simulink model "Autotrans_shift"  (R2024b)
settings: Solver=VariableStepAuto  StartTime=0.0  StopTime=35.0  FixedStep=0.001  RelTol=0.001
model workspace (MATLAB code in the model file):
  | load sldemo_autotrans_data; %load initial conditions and other necessary data
undefined symbols (not defined in the file or in its folder): converter_data, downtab, emap, Hecate_brake1, Hecate_brake2, Hecate_throttle1, Hecate_throttle2, Hecate_trans, Iei, uptab, vehicledata
(part 2 of 2)

== stateflow chart Autotrans_shift/RequirementsTable2 ==
  (default) -> (junction 1073745136)
  (junction 1073745136) -> (junction 1073745137) : {
      | % SF_REQ_REV_07
      | }
  (junction 1073745137) -> (junction 1073745139) : {
      | % ExcEvals:
      | % PriEvals:
      | }
  (junction 1073745139) -> (junction 1073745141) : {
      | % HEADER_ASSIGNMENTS
      |
      | }
  (junction 1073745141) -> (junction 1073745143) : {
      | % START_A_4
      | }
  (junction 1073745143) -> (junction 1073745145) : {
      | }
  (junction 1073745145) -> (junction 1073745147)
  (junction 1073745147) -> (junction 1073745149) : {
      | }
  (junction 1073745149) -> (junction 1073745151) : {
      | % END_A_4
      | }
  (junction 1073745151) -> (junction 1073745153) : {
      | % START_R_7
      | }
  (junction 1073745153) -> (junction 1073745155) : {
      | }
  (junction 1073745155) -> (junction 1073745157)
  (junction 1073745157) -> (junction 1073745159) [order 1] : [(((t) >= (0) && (t) <= (20)))]
  (junction 1073745157) -> (junction 1073745165) [order 2]
  (junction 1073745159) -> (junction 1073745161) : {
      | reqtable_postcondition(((speed2)/115 < 1), 'R:1');
      |
      |
      |
      |
      | }
  (junction 1073745161) -> (junction 1073745163) : {
      | }
  (junction 1073745163) -> (junction 1073745165)
  (junction 1073745165) -> (junction 1073745167)
  (junction 1073745167) -> (junction 1073745169) : {
      | % END_R_7
      | }
  (junction 1073745169) -> (junction 1073745171) : {
      | % START_R_19
      | }
  (junction 1073745171) -> (junction 1073745173) : {
      | }
  (junction 1073745173) -> (junction 1073745175)
  (junction 1073745175) -> (junction 1073745177) [order 1] : [(((t) >= (0) && (t) <= (10)))]
  (junction 1073745175) -> (junction 1073745183) [order 2]
  (junction 1073745177) -> (junction 1073745179) : {
      | reqtable_postcondition(((RPM2)/4800 < 1), 'R:2');
      |
      |
      |
      |
      | }
  (junction 1073745179) -> (junction 1073745181) : {
      | }
  (junction 1073745181) -> (junction 1073745183)
  (junction 1073745183) -> (junction 1073745185)
  (junction 1073745185) -> (junction 1073745187) : {
      | % END_R_19
      | }
  (junction 1073745187) -> (junction 1073745189) : {
      | % START_R_34
      | }
  (junction 1073745189) -> (junction 1073745191) : {
      | }
  (junction 1073745191) -> (junction 1073745193)
  (junction 1073745193) -> (junction 1073745195) [order 1] : [((t)== 0)]
  (junction 1073745193) -> (junction 1073745201) [order 2]
  (junction 1073745195) -> (junction 1073745197) : {
      | flaga_out = true;
      | flagb_out = true;
      | flagc_out = true;
      |
      | }
  (junction 1073745197) -> (junction 1073745199) : {
      | }
  (junction 1073745199) -> (junction 1073745201)
  (junction 1073745201) -> (junction 1073745203)
  (junction 1073745203) -> (junction 1073745205) : {
      | % END_R_34
      | }
  (junction 1073745205) -> (junction 1073745207) : {
      | % START_R_22
      | }
  (junction 1073745207) -> (junction 1073745209) : {
      | }
  (junction 1073745209) -> (junction 1073745211)
  (junction 1073745211) -> (junction 1073745213) [order 1] : [(((t) <= (4))) && (speed1 >= 35)]
  (junction 1073745211) -> (junction 1073745219) [order 2]
  (junction 1073745213) -> (junction 1073745215) : {
      | flaga_out = false
      |
      |
      |
      | }
  (junction 1073745215) -> (junction 1073745217) : {
      | }
  (junction 1073745217) -> (junction 1073745219)
  (junction 1073745219) -> (junction 1073745221)
  (junction 1073745221) -> (junction 1073745223) : {
      | % END_R_22
      | }
  (junction 1073745223) -> (junction 1073745225) : {
      | % START_R_67
      | }
  (junction 1073745225) -> (junction 1073745227) : {
      | }
  (junction 1073745227) -> (junction 1073745229)
  (junction 1073745229) -> (junction 1073745231) [order 1] : [((t)> 4 || ((t)> 0 && speed1 < 35))]
  (junction 1073745229) -> (junction 1073745237) [order 2]
  (junction 1073745231) -> (junction 1073745233) : {
      | flaga_out = prev(flaga_out);
      |
      |
      |
      | }
  (junction 1073745233) -> (junction 1073745235) : {
      | }
  (junction 1073745235) -> (junction 1073745237)
  (junction 1073745237) -> (junction 1073745239)
  (junction 1073745239) -> (junction 1073745241) : {
      | % END_R_67
      | }
  (junction 1073745241) -> (junction 1073745243) : {
      | % START_R_52
      | }
  (junction 1073745243) -> (junction 1073745245) : {
      | }
  (junction 1073745245) -> (junction 1073745247)
  (junction 1073745247) -> (junction 1073745249) [order 1] : [duration((((t) <= (30))) && (RPM1 < 3000)) >= 30]
  (junction 1073745247) -> (junction 1073745255) [order 2]
  (junction 1073745249) -> (junction 1073745251) : {
      | reqtable_postcondition((((flaga_in) == (true))), 'R:6');
      |
      |
      |
      |
      | }
  (junction 1073745251) -> (junction 1073745253) : {
      | }
  (junction 1073745253) -> (junction 1073745255)
  (junction 1073745255) -> (junction 1073745257)
  (junction 1073745257) -> (junction 1073745259) : {
      | % END_R_52
      | }
  (junction 1073745259) -> (junction 1073745261) : {
      | % START_R_16
      | }
  (junction 1073745261) -> (junction 1073745263) : {
      | }
  (junction 1073745263) -> (junction 1073745265)
  (junction 1073745265) -> (junction 1073745267) [order 1] : [(((t) <= (8))) && (speed1 >= 52)]
  (junction 1073745265) -> (junction 1073745273) [order 2]
  (junction 1073745267) -> (junction 1073745269) : {
      |
      | flagb_out = false;
      |
      |
      | }
  (junction 1073745269) -> (junction 1073745271) : {
      | }
  (junction 1073745271) -> (junction 1073745273)
  (junction 1073745273) -> (junction 1073745275)
  (junction 1073745275) -> (junction 1073745277) : {
      | % END_R_16
      | }
  (junction 1073745277) -> (junction 1073745279) : {
      | % START_R_70
      | }
  (junction 1073745279) -> (junction 1073745281) : {
      | }
  (junction 1073745281) -> (junction 1073745283)
  (junction 1073745283) -> (junction 1073745285) [order 1] : [((t)> 8 || ((t)> 0 && speed1 < 52))]
  (junction 1073745283) -> (junction 1073745291) [order 2]
  (junction 1073745285) -> (junction 1073745287) : {
      |
      | flagb_out = prev(flagb_out);
      |
      |
      | }
  (junction 1073745287) -> (junction 1073745289) : {
      | }
  (junction 1073745289) -> (junction 1073745291)
  (junction 1073745291) -> (junction 1073745293)
  (junction 1073745293) -> (junction 1073745295) : {
      | % END_R_70
      | }
  (junction 1073745295) -> (junction 1073745297) : {
      | % START_R_55
      | }
  (junction 1073745297) -> (junction 1073745299) : {
      | }
  (junction 1073745299) -> (junction 1073745301)
  (junction 1073745301) -> (junction 1073745303) [order 1] : [duration((((t) <= (30))) && (RPM1 < 2900)) >= 30]
  (junction 1073745301) -> (junction 1073745309) [order 2]
  (junction 1073745303) -> (junction 1073745305) : {
      | reqtable_postcondition((((flagb_in) == (true))), 'R:9');
      |
      |
      |
      |
      | }
  (junction 1073745305) -> (junction 1073745307) : {
      | }
  (junction 1073745307) -> (junction 1073745309)
  (junction 1073745309) -> (junction 1073745311)
  (junction 1073745311) -> (junction 1073745313) : {
      | % END_R_55
      | }
  (junction 1073745313) -> (junction 1073745315) : {
      | % START_R_28
      | }
  (junction 1073745315) -> (junction 1073745317) : {
      | }
  (junction 1073745317) -> (junction 1073745319)
  (junction 1073745319) -> (junction 1073745321) [order 1] : [(((t) <= (20))) && (speed1 >= 65)]
  (junction 1073745319) -> (junction 1073745327) [order 2]
  (junction 1073745321) -> (junction 1073745323) : {
      |
      |
      | flagc_out = false;
      |
      | }
  (junction 1073745323) -> (junction 1073745325) : {
      | }
  (junction 1073745325) -> (junction 1073745327)
  (junction 1073745327) -> (junction 1073745329)
  (junction 1073745329) -> (junction 1073745331) : {
      | % END_R_28
      | }
  (junction 1073745331) -> (junction 1073745333) : {
      | % START_R_73
      | }
  (junction 1073745333) -> (junction 1073745335) : {
      | }
  (junction 1073745335) -> (junction 1073745337)
  (junction 1073745337) -> (junction 1073745339) [order 1] : [((t)> 20 || ((t)> 0 && speed1 < 65))]
  (junction 1073745337) -> (junction 1073745345) [order 2]
  (junction 1073745339) -> (junction 1073745341) : {
      |
      |
      | flagc_out = prev(flagc_out);
      |
      | }
  (junction 1073745341) -> (junction 1073745343) : {
      | }
  (junction 1073745343) -> (junction 1073745345)
  (junction 1073745345) -> (junction 1073745347)
  (junction 1073745347) -> (junction 1073745349) : {
      | % END_R_73
      | }
  (junction 1073745349) -> (junction 1073745351) : {
      | % START_R_58
      | }
  (junction 1073745351) -> (junction 1073745353) : {
      | }
  (junction 1073745353) -> (junction 1073745355)
  (junction 1073745355) -> (junction 1073745357) [order 1] : [duration((((t) <= (30))) && (RPM1 < 3000)) >= 30]
  (junction 1073745355) -> (junction 1073745363) [order 2]
  (junction 1073745357) -> (junction 1073745359) : {
      | reqtable_postcondition((((flagc_in) == (true))), 'R:12');
      |
      |
      |
      |
      | }
  (junction 1073745359) -> (junction 1073745361) : {
      | }
  (junction 1073745361) -> (junction 1073745363)
  (junction 1073745363) -> (junction 1073745365)
  (junction 1073745365) -> (junction 1073745367) : {
      | % END_R_58
      | }
  (junction 1073745367) -> (junction 1073745369) : {
      | % START_R_61
      | }
  (junction 1073745369) -> (junction 1073745371) : {
      | }
  (junction 1073745371) -> (junction 1073745373)
  (junction 1073745373) -> (junction 1073745375) [order 1] : [(((t) >= (0) && (t) <= (50)))]
  (junction 1073745373) -> (junction 1073745381) [order 2]
  (junction 1073745375) -> (junction 1073745377) : {
      | reqtable_postcondition((((speed2) >= (0))) && (((RPM2) >= (0))) && ((flaga_in)== true ||(flaga_in)== false) && ((flagb_in)== true ||(flagb_in)== false) && ((flagc_in)== true ||(flagc_in)== false), 'R:13');
      |
      |
      |
      |
      | }
  (junction 1073745377) -> (junction 1073745379) : {
      | }
  (junction 1073745379) -> (junction 1073745381)
  (junction 1073745381) -> (junction 1073745383)
  (junction 1073745383) -> (junction 1073745385) : {
      | % END_R_61
      | }
  data: RPM1 input; RPM2 input; speed1 input; speed2 input; flaga_out output boolean =true; flagc_out output boolean =true; flagb_out output boolean =true; flaga_in input boolean; flagc_in input boolean; flagb_in input boolean

== stateflow chart Autotrans_shift/RequirementsTable3 ==
  (default) -> (junction 1073745136)
  (junction 1073745136) -> (junction 1073745137) : {
      | % SF_REQ_REV_07
      | }
  (junction 1073745137) -> (junction 1073745139) : {
      | % ExcEvals:
      | % PriEvals:
      | }
  (junction 1073745139) -> (junction 1073745141) : {
      | % HEADER_ASSIGNMENTS
      |
      | }
  (junction 1073745141) -> (junction 1073745143) : {
      | % START_A_4
      | }
  (junction 1073745143) -> (junction 1073745145) : {
      | }
  (junction 1073745145) -> (junction 1073745147)
  (junction 1073745147) -> (junction 1073745149) : {
      | }
  (junction 1073745149) -> (junction 1073745151) : {
      | % END_A_4
      | }
  (junction 1073745151) -> (junction 1073745153) : {
      | % START_R_7
      | }
  (junction 1073745153) -> (junction 1073745155) : {
      | }
  (junction 1073745155) -> (junction 1073745157)
  (junction 1073745157) -> (junction 1073745159) [order 1] : [(((t) >= (0) && (t) <= (25)))]
  (junction 1073745157) -> (junction 1073745165) [order 2]
  (junction 1073745159) -> (junction 1073745161) : {
      | reqtable_postcondition(((speed2)/125 < 1), 'R:1');
      |
      |
      |
      |
      | }
  (junction 1073745161) -> (junction 1073745163) : {
      | }
  (junction 1073745163) -> (junction 1073745165)
  (junction 1073745165) -> (junction 1073745167)
  (junction 1073745167) -> (junction 1073745169) : {
      | % END_R_7
      | }
  (junction 1073745169) -> (junction 1073745171) : {
      | % START_R_19
      | }
  (junction 1073745171) -> (junction 1073745173) : {
      | }
  (junction 1073745173) -> (junction 1073745175)
  (junction 1073745175) -> (junction 1073745177) [order 1] : [(((t) >= (0) && (t) <= (10)))]
  (junction 1073745175) -> (junction 1073745183) [order 2]
  (junction 1073745177) -> (junction 1073745179) : {
      | reqtable_postcondition(((RPM2)/4800 < 1), 'R:2');
      |
      |
      |
      |
      | }
  (junction 1073745179) -> (junction 1073745181) : {
      | }
  (junction 1073745181) -> (junction 1073745183)
  (junction 1073745183) -> (junction 1073745185)
  (junction 1073745185) -> (junction 1073745187) : {
      | % END_R_19
      | }
  (junction 1073745187) -> (junction 1073745189) : {
      | % START_R_34
      | }
  (junction 1073745189) -> (junction 1073745191) : {
      | }
  (junction 1073745191) -> (junction 1073745193)
  (junction 1073745193) -> (junction 1073745195) [order 1] : [((t)== 0)]
  (junction 1073745193) -> (junction 1073745201) [order 2]
  (junction 1073745195) -> (junction 1073745197) : {
      | flaga_out = true;
      | flagb_out = true;
      | flagc_out = true;
      |
      | }
  (junction 1073745197) -> (junction 1073745199) : {
      | }
  (junction 1073745199) -> (junction 1073745201)
  (junction 1073745201) -> (junction 1073745203)
  (junction 1073745203) -> (junction 1073745205) : {
      | % END_R_34
      | }
  (junction 1073745205) -> (junction 1073745207) : {
      | % START_R_22
      | }
  (junction 1073745207) -> (junction 1073745209) : {
      | }
  (junction 1073745209) -> (junction 1073745211)
  (junction 1073745211) -> (junction 1073745213) [order 1] : [(((t) <= (4))) && (speed1 >= 35)]
  (junction 1073745211) -> (junction 1073745219) [order 2]
  (junction 1073745213) -> (junction 1073745215) : {
      | flaga_out = false
      |
      |
      |
      | }
  (junction 1073745215) -> (junction 1073745217) : {
      | }
  (junction 1073745217) -> (junction 1073745219)
  (junction 1073745219) -> (junction 1073745221)
  (junction 1073745221) -> (junction 1073745223) : {
      | % END_R_22
      | }
  (junction 1073745223) -> (junction 1073745225) : {
      | % START_R_67
      | }
  (junction 1073745225) -> (junction 1073745227) : {
      | }
  (junction 1073745227) -> (junction 1073745229)
  (junction 1073745229) -> (junction 1073745231) [order 1] : [((t)> 4 || ((t)> 0 && speed1 < 35))]
  (junction 1073745229) -> (junction 1073745237) [order 2]
  (junction 1073745231) -> (junction 1073745233) : {
      | flaga_out = prev(flaga_out);
      |
      |
      |
      | }
  (junction 1073745233) -> (junction 1073745235) : {
      | }
  (junction 1073745235) -> (junction 1073745237)
  (junction 1073745237) -> (junction 1073745239)
  (junction 1073745239) -> (junction 1073745241) : {
      | % END_R_67
      | }
  (junction 1073745241) -> (junction 1073745243) : {
      | % START_R_52
      | }
  (junction 1073745243) -> (junction 1073745245) : {
      | }
  (junction 1073745245) -> (junction 1073745247)
  (junction 1073745247) -> (junction 1073745249) [order 1] : [duration((((t) <= (30))) && (RPM1 < 3000)) >= 30]
  (junction 1073745247) -> (junction 1073745255) [order 2]
  (junction 1073745249) -> (junction 1073745251) : {
      | reqtable_postcondition((((flaga_in) == (true))), 'R:6');
      |
      |
      |
      |
      | }
  (junction 1073745251) -> (junction 1073745253) : {
      | }
  (junction 1073745253) -> (junction 1073745255)
  (junction 1073745255) -> (junction 1073745257)
  (junction 1073745257) -> (junction 1073745259) : {
      | % END_R_52
      | }
  (junction 1073745259) -> (junction 1073745261) : {
      | % START_R_16
      | }
  (junction 1073745261) -> (junction 1073745263) : {
      | }
  (junction 1073745263) -> (junction 1073745265)
  (junction 1073745265) -> (junction 1073745267) [order 1] : [(((t) <= (8))) && (speed1 >= 50)]
  (junction 1073745265) -> (junction 1073745273) [order 2]
  (junction 1073745267) -> (junction 1073745269) : {
      |
      | flagb_out = false;
      |
      |
      | }
  (junction 1073745269) -> (junction 1073745271) : {
      | }
  (junction 1073745271) -> (junction 1073745273)
  (junction 1073745273) -> (junction 1073745275)
  (junction 1073745275) -> (junction 1073745277) : {
      | % END_R_16
      | }
  (junction 1073745277) -> (junction 1073745279) : {
      | % START_R_70
      | }
  (junction 1073745279) -> (junction 1073745281) : {
      | }
  (junction 1073745281) -> (junction 1073745283)
  (junction 1073745283) -> (junction 1073745285) [order 1] : [((t)> 8 || ((t)> 0 && speed1 < 50))]
  (junction 1073745283) -> (junction 1073745291) [order 2]
  (junction 1073745285) -> (junction 1073745287) : {
      |
      | flagb_out = prev(flagb_out);
      |
      |
      | }
  (junction 1073745287) -> (junction 1073745289) : {
      | }
  (junction 1073745289) -> (junction 1073745291)
  (junction 1073745291) -> (junction 1073745293)
  (junction 1073745293) -> (junction 1073745295) : {
      | % END_R_70
      | }
  (junction 1073745295) -> (junction 1073745297) : {
      | % START_R_55
      | }
  (junction 1073745297) -> (junction 1073745299) : {
      | }
  (junction 1073745299) -> (junction 1073745301)
  (junction 1073745301) -> (junction 1073745303) [order 1] : [duration((((t) <= (30))) && (RPM1 < 3000)) >= 30]
  (junction 1073745301) -> (junction 1073745309) [order 2]
  (junction 1073745303) -> (junction 1073745305) : {
      | reqtable_postcondition((((flagb_in) == (true))), 'R:9');
      |
      |
      |
      |
      | }
  (junction 1073745305) -> (junction 1073745307) : {
      | }
  (junction 1073745307) -> (junction 1073745309)
  (junction 1073745309) -> (junction 1073745311)
  (junction 1073745311) -> (junction 1073745313) : {
      | % END_R_55
      | }
  (junction 1073745313) -> (junction 1073745315) : {
      | % START_R_28
      | }
  (junction 1073745315) -> (junction 1073745317) : {
      | }
  (junction 1073745317) -> (junction 1073745319)
  (junction 1073745319) -> (junction 1073745321) [order 1] : [(((t) <= (20))) && (speed1 >= 67)]
  (junction 1073745319) -> (junction 1073745327) [order 2]
  (junction 1073745321) -> (junction 1073745323) : {
      |
      |
      | flagc_out = false;
      |
      | }
  (junction 1073745323) -> (junction 1073745325) : {
      | }
  (junction 1073745325) -> (junction 1073745327)
  (junction 1073745327) -> (junction 1073745329)
  (junction 1073745329) -> (junction 1073745331) : {
      | % END_R_28
      | }
  (junction 1073745331) -> (junction 1073745333) : {
      | % START_R_73
      | }
  (junction 1073745333) -> (junction 1073745335) : {
      | }
  (junction 1073745335) -> (junction 1073745337)
  (junction 1073745337) -> (junction 1073745339) [order 1] : [((t)> 20 || ((t)> 0 && speed1 < 67))]
  (junction 1073745337) -> (junction 1073745345) [order 2]
  (junction 1073745339) -> (junction 1073745341) : {
      |
      |
      | flagc_out = prev(flagc_out);
      |
      | }
  (junction 1073745341) -> (junction 1073745343) : {
      | }
  (junction 1073745343) -> (junction 1073745345)
  (junction 1073745345) -> (junction 1073745347)
  (junction 1073745347) -> (junction 1073745349) : {
      | % END_R_73
      | }
  (junction 1073745349) -> (junction 1073745351) : {
      | % START_R_58
      | }
  (junction 1073745351) -> (junction 1073745353) : {
      | }
  (junction 1073745353) -> (junction 1073745355)
  (junction 1073745355) -> (junction 1073745357) [order 1] : [duration((((t) <= (30))) && (RPM1 < 2900)) >= 30]
  (junction 1073745355) -> (junction 1073745363) [order 2]
  (junction 1073745357) -> (junction 1073745359) : {
      | reqtable_postcondition((((flagc_in) == (true))), 'R:12');
      |
      |
      |
      |
      | }
  (junction 1073745359) -> (junction 1073745361) : {
      | }
  (junction 1073745361) -> (junction 1073745363)
  (junction 1073745363) -> (junction 1073745365)
  (junction 1073745365) -> (junction 1073745367) : {
      | % END_R_58
      | }
  (junction 1073745367) -> (junction 1073745369) : {
      | % START_R_61
      | }
  (junction 1073745369) -> (junction 1073745371) : {
      | }
  (junction 1073745371) -> (junction 1073745373)
  (junction 1073745373) -> (junction 1073745375) [order 1] : [(((t) >= (0) && (t) <= (50)))]
  (junction 1073745373) -> (junction 1073745381) [order 2]
  (junction 1073745375) -> (junction 1073745377) : {
      | reqtable_postcondition((((speed2) >= (0))) && (((RPM2) >= (0))) && ((flaga_in)== true ||(flaga_in)== false) && ((flagb_in)== true ||(flagb_in)== false) && ((flagc_in)== true ||(flagc_in)== false), 'R:13');
      |
      |
      |
      |
      | }
  (junction 1073745377) -> (junction 1073745379) : {
      | }
  (junction 1073745379) -> (junction 1073745381)
  (junction 1073745381) -> (junction 1073745383)
  (junction 1073745383) -> (junction 1073745385) : {
      | % END_R_61
      | }
  data: RPM1 input; RPM2 input; speed1 input; speed2 input; flaga_out output boolean =true; flagc_out output boolean =true; flagb_out output boolean =true; flaga_in input boolean; flagc_in input boolean; flagb_in input boolean

== stateflow chart Autotrans_shift/RequirementsTable4 ==
  (default) -> (junction 1073745136)
  (junction 1073745136) -> (junction 1073745137) : {
      | % SF_REQ_REV_07
      | }
  (junction 1073745137) -> (junction 1073745139) : {
      | % ExcEvals:
      | % PriEvals:
      | }
  (junction 1073745139) -> (junction 1073745141) : {
      | % HEADER_ASSIGNMENTS
      |
      | }
  (junction 1073745141) -> (junction 1073745143) : {
      | % START_A_4
      | }
  (junction 1073745143) -> (junction 1073745145) : {
      | }
  (junction 1073745145) -> (junction 1073745147)
  (junction 1073745147) -> (junction 1073745149) : {
      | }
  (junction 1073745149) -> (junction 1073745151) : {
      | % END_A_4
      | }
  (junction 1073745151) -> (junction 1073745153) : {
      | % START_R_7
      | }
  (junction 1073745153) -> (junction 1073745155) : {
      | }
  (junction 1073745155) -> (junction 1073745157)
  (junction 1073745157) -> (junction 1073745159) [order 1] : [(((t) >= (0) && (t) <= (25)))]
  (junction 1073745157) -> (junction 1073745165) [order 2]
  (junction 1073745159) -> (junction 1073745161) : {
      | reqtable_postcondition(((speed2)/125 < 1), 'R:1');
      |
      |
      |
      |
      | }
  (junction 1073745161) -> (junction 1073745163) : {
      | }
  (junction 1073745163) -> (junction 1073745165)
  (junction 1073745165) -> (junction 1073745167)
  (junction 1073745167) -> (junction 1073745169) : {
      | % END_R_7
      | }
  (junction 1073745169) -> (junction 1073745171) : {
      | % START_R_19
      | }
  (junction 1073745171) -> (junction 1073745173) : {
      | }
  (junction 1073745173) -> (junction 1073745175)
  (junction 1073745175) -> (junction 1073745177) [order 1] : [(((t) >= (0) && (t) <= (8)))]
  (junction 1073745175) -> (junction 1073745183) [order 2]
  (junction 1073745177) -> (junction 1073745179) : {
      | reqtable_postcondition(((RPM2)/4750 < 1), 'R:2');
      |
      |
      |
      |
      | }
  (junction 1073745179) -> (junction 1073745181) : {
      | }
  (junction 1073745181) -> (junction 1073745183)
  (junction 1073745183) -> (junction 1073745185)
  (junction 1073745185) -> (junction 1073745187) : {
      | % END_R_19
      | }
  (junction 1073745187) -> (junction 1073745189) : {
      | % START_R_34
      | }
  (junction 1073745189) -> (junction 1073745191) : {
      | }
  (junction 1073745191) -> (junction 1073745193)
  (junction 1073745193) -> (junction 1073745195) [order 1] : [((t)== 0)]
  (junction 1073745193) -> (junction 1073745201) [order 2]
  (junction 1073745195) -> (junction 1073745197) : {
      | flaga_out = true;
      | flagb_out = true;
      | flagc_out = true;
      |
      | }
  (junction 1073745197) -> (junction 1073745199) : {
      | }
  (junction 1073745199) -> (junction 1073745201)
  (junction 1073745201) -> (junction 1073745203)
  (junction 1073745203) -> (junction 1073745205) : {
      | % END_R_34
      | }
  (junction 1073745205) -> (junction 1073745207) : {
      | % START_R_22
      | }
  (junction 1073745207) -> (junction 1073745209) : {
      | }
  (junction 1073745209) -> (junction 1073745211)
  (junction 1073745211) -> (junction 1073745213) [order 1] : [(((t) <= (4))) && (speed1 >= 32)]
  (junction 1073745211) -> (junction 1073745219) [order 2]
  (junction 1073745213) -> (junction 1073745215) : {
      | flaga_out = false
      |
      |
      |
      | }
  (junction 1073745215) -> (junction 1073745217) : {
      | }
  (junction 1073745217) -> (junction 1073745219)
  (junction 1073745219) -> (junction 1073745221)
  (junction 1073745221) -> (junction 1073745223) : {
      | % END_R_22
      | }
  (junction 1073745223) -> (junction 1073745225) : {
      | % START_R_67
      | }
  (junction 1073745225) -> (junction 1073745227) : {
      | }
  (junction 1073745227) -> (junction 1073745229)
  (junction 1073745229) -> (junction 1073745231) [order 1] : [((t)> 4 || ((t)> 0 && speed1 < 32))]
  (junction 1073745229) -> (junction 1073745237) [order 2]
  (junction 1073745231) -> (junction 1073745233) : {
      | flaga_out = prev(flaga_out);
      |
      |
      |
      | }
  (junction 1073745233) -> (junction 1073745235) : {
      | }
  (junction 1073745235) -> (junction 1073745237)
  (junction 1073745237) -> (junction 1073745239)
  (junction 1073745239) -> (junction 1073745241) : {
      | % END_R_67
      | }
  (junction 1073745241) -> (junction 1073745243) : {
      | % START_R_52
      | }
  (junction 1073745243) -> (junction 1073745245) : {
      | }
  (junction 1073745245) -> (junction 1073745247)
  (junction 1073745247) -> (junction 1073745249) [order 1] : [duration((((t) <= (30))) && (RPM1 < 2900)) >= 30]
  (junction 1073745247) -> (junction 1073745255) [order 2]
  (junction 1073745249) -> (junction 1073745251) : {
      | reqtable_postcondition((((flaga_in) == (true))), 'R:6');
      |
      |
      |
      |
      | }
  (junction 1073745251) -> (junction 1073745253) : {
      | }
  (junction 1073745253) -> (junction 1073745255)
  (junction 1073745255) -> (junction 1073745257)
  (junction 1073745257) -> (junction 1073745259) : {
      | % END_R_52
      | }
  (junction 1073745259) -> (junction 1073745261) : {
      | % START_R_16
      | }
  (junction 1073745261) -> (junction 1073745263) : {
      | }
  (junction 1073745263) -> (junction 1073745265)
  (junction 1073745265) -> (junction 1073745267) [order 1] : [(((t) <= (8))) && (speed1 >= 52)]
  (junction 1073745265) -> (junction 1073745273) [order 2]
  (junction 1073745267) -> (junction 1073745269) : {
      |
      | flagb_out = false;
      |
      |
      | }
  (junction 1073745269) -> (junction 1073745271) : {
      | }
  (junction 1073745271) -> (junction 1073745273)
  (junction 1073745273) -> (junction 1073745275)
  (junction 1073745275) -> (junction 1073745277) : {
      | % END_R_16
      | }
  (junction 1073745277) -> (junction 1073745279) : {
      | % START_R_70
      | }
  (junction 1073745279) -> (junction 1073745281) : {
      | }
  (junction 1073745281) -> (junction 1073745283)
  (junction 1073745283) -> (junction 1073745285) [order 1] : [((t)> 8 || ((t)> 0 && speed1 < 52))]
  (junction 1073745283) -> (junction 1073745291) [order 2]
  (junction 1073745285) -> (junction 1073745287) : {
      |
      | flagb_out = prev(flagb_out);
      |
      |
      | }
  (junction 1073745287) -> (junction 1073745289) : {
      | }
  (junction 1073745289) -> (junction 1073745291)
  (junction 1073745291) -> (junction 1073745293)
  (junction 1073745293) -> (junction 1073745295) : {
      | % END_R_70
      | }
  (junction 1073745295) -> (junction 1073745297) : {
      | % START_R_55
      | }
  (junction 1073745297) -> (junction 1073745299) : {
      | }
  (junction 1073745299) -> (junction 1073745301)
  (junction 1073745301) -> (junction 1073745303) [order 1] : [duration((((t) <= (30))) && (RPM1 < 2900)) >= 30]
  (junction 1073745301) -> (junction 1073745309) [order 2]
  (junction 1073745303) -> (junction 1073745305) : {
      | reqtable_postcondition((((flagb_in) == (true))), 'R:9');
      |
      |
      |
      |
      | }
  (junction 1073745305) -> (junction 1073745307) : {
      | }
  (junction 1073745307) -> (junction 1073745309)
  (junction 1073745309) -> (junction 1073745311)
  (junction 1073745311) -> (junction 1073745313) : {
      | % END_R_55
      | }
  (junction 1073745313) -> (junction 1073745315) : {
      | % START_R_28
      | }
  (junction 1073745315) -> (junction 1073745317) : {
      | }
  (junction 1073745317) -> (junction 1073745319)
  (junction 1073745319) -> (junction 1073745321) [order 1] : [(((t) <= (20))) && (speed1 >= 67)]
  (junction 1073745319) -> (junction 1073745327) [order 2]
  (junction 1073745321) -> (junction 1073745323) : {
      |
      |
      | flagc_out = false;
      |
      | }
  (junction 1073745323) -> (junction 1073745325) : {
      | }
  (junction 1073745325) -> (junction 1073745327)
  (junction 1073745327) -> (junction 1073745329)
  (junction 1073745329) -> (junction 1073745331) : {
      | % END_R_28
      | }
  (junction 1073745331) -> (junction 1073745333) : {
      | % START_R_73
      | }
  (junction 1073745333) -> (junction 1073745335) : {
      | }
  (junction 1073745335) -> (junction 1073745337)
  (junction 1073745337) -> (junction 1073745339) [order 1] : [((t)> 20 || ((t)> 0 && speed1 < 67))]
  (junction 1073745337) -> (junction 1073745345) [order 2]
  (junction 1073745339) -> (junction 1073745341) : {
      |
      |
      | flagc_out = prev(flagc_out);
      |
      | }
  (junction 1073745341) -> (junction 1073745343) : {
      | }
  (junction 1073745343) -> (junction 1073745345)
  (junction 1073745345) -> (junction 1073745347)
  (junction 1073745347) -> (junction 1073745349) : {
      | % END_R_73
      | }
  (junction 1073745349) -> (junction 1073745351) : {
      | % START_R_58
      | }
  (junction 1073745351) -> (junction 1073745353) : {
      | }
  (junction 1073745353) -> (junction 1073745355)
  (junction 1073745355) -> (junction 1073745357) [order 1] : [duration((((t) <= (30))) && (RPM1 < 2900)) >= 30]
  (junction 1073745355) -> (junction 1073745363) [order 2]
  (junction 1073745357) -> (junction 1073745359) : {
      | reqtable_postcondition((((flagc_in) == (true))), 'R:12');
      |
      |
      |
      |
      | }
  (junction 1073745359) -> (junction 1073745361) : {
      | }
  (junction 1073745361) -> (junction 1073745363)
  (junction 1073745363) -> (junction 1073745365)
  (junction 1073745365) -> (junction 1073745367) : {
      | % END_R_58
      | }
  (junction 1073745367) -> (junction 1073745369) : {
      | % START_R_61
      | }
  (junction 1073745369) -> (junction 1073745371) : {
      | }
  (junction 1073745371) -> (junction 1073745373)
  (junction 1073745373) -> (junction 1073745375) [order 1] : [(((t) >= (0) && (t) <= (50)))]
  (junction 1073745373) -> (junction 1073745381) [order 2]
  (junction 1073745375) -> (junction 1073745377) : {
      | reqtable_postcondition((((speed2) >= (0))) && (((RPM2) >= (0))) && ((flaga_in)== true ||(flaga_in)== false) && ((flagb_in)== true ||(flagb_in)== false) && ((flagc_in)== true ||(flagc_in)== false), 'R:13');
      |
      |
      |
      |
      | }
  (junction 1073745377) -> (junction 1073745379) : {
      | }
  (junction 1073745379) -> (junction 1073745381)
  (junction 1073745381) -> (junction 1073745383)
  (junction 1073745383) -> (junction 1073745385) : {
      | % END_R_61
      | }
  data: RPM1 input; RPM2 input; speed1 input; speed2 input; flaga_out output boolean =true; flagc_out output boolean =true; flagb_out output boolean =true; flaga_in input boolean; flagc_in input boolean; flagb_in input boolean

== stateflow chart Autotrans_shift/RequirementsTable5 ==
  (default) -> (junction 1073745136)
  (junction 1073745136) -> (junction 1073745137) : {
      | % SF_REQ_REV_07
      | }
  (junction 1073745137) -> (junction 1073745139) : {
      | % ExcEvals:
      | % PriEvals:
      | }
  (junction 1073745139) -> (junction 1073745141) : {
      | % HEADER_ASSIGNMENTS
      |
      | }
  (junction 1073745141) -> (junction 1073745143) : {
      | % START_A_4
      | }
  (junction 1073745143) -> (junction 1073745145) : {
      | }
  (junction 1073745145) -> (junction 1073745147)
  (junction 1073745147) -> (junction 1073745149) : {
      | }
  (junction 1073745149) -> (junction 1073745151) : {
      | % END_A_4
      | }
  (junction 1073745151) -> (junction 1073745153) : {
      | % START_R_7
      | }
  (junction 1073745153) -> (junction 1073745155) : {
      | }
  (junction 1073745155) -> (junction 1073745157)
  (junction 1073745157) -> (junction 1073745159) [order 1] : [(((t) >= (0) && (t) <= (25)))]
  (junction 1073745157) -> (junction 1073745165) [order 2]
  (junction 1073745159) -> (junction 1073745161) : {
      | reqtable_postcondition(((speed2)/125 < 1), 'R:1');
      |
      |
      |
      |
      | }
  (junction 1073745161) -> (junction 1073745163) : {
      | }
  (junction 1073745163) -> (junction 1073745165)
  (junction 1073745165) -> (junction 1073745167)
  (junction 1073745167) -> (junction 1073745169) : {
      | % END_R_7
      | }
  (junction 1073745169) -> (junction 1073745171) : {
      | % START_R_19
      | }
  (junction 1073745171) -> (junction 1073745173) : {
      | }
  (junction 1073745173) -> (junction 1073745175)
  (junction 1073745175) -> (junction 1073745177) [order 1] : [(((t) >= (0) && (t) <= (8)))]
  (junction 1073745175) -> (junction 1073745183) [order 2]
  (junction 1073745177) -> (junction 1073745179) : {
      | reqtable_postcondition(((RPM2)/4750 < 1), 'R:2');
      |
      |
      |
      |
      | }
  (junction 1073745179) -> (junction 1073745181) : {
      | }
  (junction 1073745181) -> (junction 1073745183)
  (junction 1073745183) -> (junction 1073745185)
  (junction 1073745185) -> (junction 1073745187) : {
      | % END_R_19
      | }
  (junction 1073745187) -> (junction 1073745189) : {
      | % START_R_34
      | }
  (junction 1073745189) -> (junction 1073745191) : {
      | }
  (junction 1073745191) -> (junction 1073745193)
  (junction 1073745193) -> (junction 1073745195) [order 1] : [((t)== 0)]
  (junction 1073745193) -> (junction 1073745201) [order 2]
  (junction 1073745195) -> (junction 1073745197) : {
      | flaga_out = true;
      | flagb_out = true;
      | flagc_out = true;
      |
      | }
  (junction 1073745197) -> (junction 1073745199) : {
      | }
  (junction 1073745199) -> (junction 1073745201)
  (junction 1073745201) -> (junction 1073745203)
  (junction 1073745203) -> (junction 1073745205) : {
      | % END_R_34
      | }
  (junction 1073745205) -> (junction 1073745207) : {
      | % START_R_22
      | }
  (junction 1073745207) -> (junction 1073745209) : {
      | }
  (junction 1073745209) -> (junction 1073745211)
  (junction 1073745211) -> (junction 1073745213) [order 1] : [(((t) <= (5))) && (speed1 >= 35)]
  (junction 1073745211) -> (junction 1073745219) [order 2]
  (junction 1073745213) -> (junction 1073745215) : {
      | flaga_out = false
      |
      |
      |
      | }
  (junction 1073745215) -> (junction 1073745217) : {
      | }
  (junction 1073745217) -> (junction 1073745219)
  (junction 1073745219) -> (junction 1073745221)
  (junction 1073745221) -> (junction 1073745223) : {
      | % END_R_22
      | }
  (junction 1073745223) -> (junction 1073745225) : {
      | % START_R_67
      | }
  (junction 1073745225) -> (junction 1073745227) : {
      | }
  (junction 1073745227) -> (junction 1073745229)
  (junction 1073745229) -> (junction 1073745231) [order 1] : [((t)> 5 || ((t)> 0 && speed1 < 35))]
  (junction 1073745229) -> (junction 1073745237) [order 2]
  (junction 1073745231) -> (junction 1073745233) : {
      | flaga_out = prev(flaga_out);
      |
      |
      |
      | }
  (junction 1073745233) -> (junction 1073745235) : {
      | }
  (junction 1073745235) -> (junction 1073745237)
  (junction 1073745237) -> (junction 1073745239)
  (junction 1073745239) -> (junction 1073745241) : {
      | % END_R_67
      | }
  (junction 1073745241) -> (junction 1073745243) : {
      | % START_R_52
      | }
  (junction 1073745243) -> (junction 1073745245) : {
      | }
  (junction 1073745245) -> (junction 1073745247)
  (junction 1073745247) -> (junction 1073745249) [order 1] : [duration((((t) <= (30))) && (RPM1 < 3000)) >= 30]
  (junction 1073745247) -> (junction 1073745255) [order 2]
  (junction 1073745249) -> (junction 1073745251) : {
      | reqtable_postcondition((((flaga_in) == (true))), 'R:6');
      |
      |
      |
      |
      | }
  (junction 1073745251) -> (junction 1073745253) : {
      | }
  (junction 1073745253) -> (junction 1073745255)
  (junction 1073745255) -> (junction 1073745257)
  (junction 1073745257) -> (junction 1073745259) : {
      | % END_R_52
      | }
  (junction 1073745259) -> (junction 1073745261) : {
      | % START_R_16
      | }
  (junction 1073745261) -> (junction 1073745263) : {
      | }
  (junction 1073745263) -> (junction 1073745265)
  (junction 1073745265) -> (junction 1073745267) [order 1] : [(((t) <= (10))) && (speed1 >= 50)]
  (junction 1073745265) -> (junction 1073745273) [order 2]
  (junction 1073745267) -> (junction 1073745269) : {
      |
      | flagb_out = false;
      |
      |
      | }
  (junction 1073745269) -> (junction 1073745271) : {
      | }
  (junction 1073745271) -> (junction 1073745273)
  (junction 1073745273) -> (junction 1073745275)
  (junction 1073745275) -> (junction 1073745277) : {
      | % END_R_16
      | }
  (junction 1073745277) -> (junction 1073745279) : {
      | % START_R_70
      | }
  (junction 1073745279) -> (junction 1073745281) : {
      | }
  (junction 1073745281) -> (junction 1073745283)
  (junction 1073745283) -> (junction 1073745285) [order 1] : [((t)> 10 || ((t)> 0 && speed1 < 50))]
  (junction 1073745283) -> (junction 1073745291) [order 2]
  (junction 1073745285) -> (junction 1073745287) : {
      |
      | flagb_out = prev(flagb_out);
      |
      |
      | }
  (junction 1073745287) -> (junction 1073745289) : {
      | }
  (junction 1073745289) -> (junction 1073745291)
  (junction 1073745291) -> (junction 1073745293)
  (junction 1073745293) -> (junction 1073745295) : {
      | % END_R_70
      | }
  (junction 1073745295) -> (junction 1073745297) : {
      | % START_R_55
      | }
  (junction 1073745297) -> (junction 1073745299) : {
      | }
  (junction 1073745299) -> (junction 1073745301)
  (junction 1073745301) -> (junction 1073745303) [order 1] : [duration((((t) <= (30))) && (RPM1 < 3000)) >= 30]
  (junction 1073745301) -> (junction 1073745309) [order 2]
  (junction 1073745303) -> (junction 1073745305) : {
      | reqtable_postcondition((((flagb_in) == (true))), 'R:9');
      |
      |
      |
      |
      | }
  (junction 1073745305) -> (junction 1073745307) : {
      | }
  (junction 1073745307) -> (junction 1073745309)
  (junction 1073745309) -> (junction 1073745311)
  (junction 1073745311) -> (junction 1073745313) : {
      | % END_R_55
      | }
  (junction 1073745313) -> (junction 1073745315) : {
      | % START_R_28
      | }
  (junction 1073745315) -> (junction 1073745317) : {
      | }
  (junction 1073745317) -> (junction 1073745319)
  (junction 1073745319) -> (junction 1073745321) [order 1] : [(((t) <= (22))) && (speed1 >= 65)]
  (junction 1073745319) -> (junction 1073745327) [order 2]
  (junction 1073745321) -> (junction 1073745323) : {
      |
      |
      | flagc_out = false;
      |
      | }
  (junction 1073745323) -> (junction 1073745325) : {
      | }
  (junction 1073745325) -> (junction 1073745327)
  (junction 1073745327) -> (junction 1073745329)
  (junction 1073745329) -> (junction 1073745331) : {
      | % END_R_28
      | }
  (junction 1073745331) -> (junction 1073745333) : {
      | % START_R_73
      | }
  (junction 1073745333) -> (junction 1073745335) : {
      | }
  (junction 1073745335) -> (junction 1073745337)
  (junction 1073745337) -> (junction 1073745339) [order 1] : [((t)> 22 || ((t)> 0 && speed1 < 65))]
  (junction 1073745337) -> (junction 1073745345) [order 2]
  (junction 1073745339) -> (junction 1073745341) : {
      |
      |
      | flagc_out = prev(flagc_out);
      |
      | }
  (junction 1073745341) -> (junction 1073745343) : {
      | }
  (junction 1073745343) -> (junction 1073745345)
  (junction 1073745345) -> (junction 1073745347)
  (junction 1073745347) -> (junction 1073745349) : {
      | % END_R_73
      | }
  (junction 1073745349) -> (junction 1073745351) : {
      | % START_R_58
      | }
  (junction 1073745351) -> (junction 1073745353) : {
      | }
  (junction 1073745353) -> (junction 1073745355)
  (junction 1073745355) -> (junction 1073745357) [order 1] : [duration((((t) <= (30))) && (RPM1 < 3000)) >= 30]
  (junction 1073745355) -> (junction 1073745363) [order 2]
  (junction 1073745357) -> (junction 1073745359) : {
      | reqtable_postcondition((((flagc_in) == (true))), 'R:12');
      |
      |
      |
      |
      | }
  (junction 1073745359) -> (junction 1073745361) : {
      | }
  (junction 1073745361) -> (junction 1073745363)
  (junction 1073745363) -> (junction 1073745365)
  (junction 1073745365) -> (junction 1073745367) : {
      | % END_R_58
      | }
  (junction 1073745367) -> (junction 1073745369) : {
      | % START_R_61
      | }
  (junction 1073745369) -> (junction 1073745371) : {
      | }
  (junction 1073745371) -> (junction 1073745373)
  (junction 1073745373) -> (junction 1073745375) [order 1] : [(((t) >= (0) && (t) <= (50)))]
  (junction 1073745373) -> (junction 1073745381) [order 2]
  (junction 1073745375) -> (junction 1073745377) : {
      | reqtable_postcondition((((speed2) >= (0))) && (((RPM2) >= (0))) && ((flaga_in)== true ||(flaga_in)== false) && ((flagb_in)== true ||(flagb_in)== false) && ((flagc_in)== true ||(flagc_in)== false), 'R:13');
      |
      |
      |
      |
      | }
  (junction 1073745377) -> (junction 1073745379) : {
      | }
  (junction 1073745379) -> (junction 1073745381)
  (junction 1073745381) -> (junction 1073745383)
  (junction 1073745383) -> (junction 1073745385) : {
      | % END_R_61
      | }
  data: RPM1 input; RPM2 input; speed1 input; speed2 input; flaga_out output boolean =true; flagc_out output boolean =true; flagb_out output boolean =true; flaga_in input boolean; flagc_in input boolean; flagb_in input boolean

== stateflow chart Autotrans_shift/RequirementsTable ==
  (default) -> (junction 1073745136)
  (junction 1073745136) -> (junction 1073745137) : {
      | % SF_REQ_REV_07
      | }
  (junction 1073745137) -> (junction 1073745139) : {
      | % ExcEvals:
      | % PriEvals:
      | }
  (junction 1073745139) -> (junction 1073745141) : {
      | % HEADER_ASSIGNMENTS
      |
      | }
  (junction 1073745141) -> (junction 1073745143) : {
      | % START_A_4
      | }
  (junction 1073745143) -> (junction 1073745145) : {
      | }
  (junction 1073745145) -> (junction 1073745147)
  (junction 1073745147) -> (junction 1073745149) : {
      | }
  (junction 1073745149) -> (junction 1073745151) : {
      | % END_A_4
      | }
  (junction 1073745151) -> (junction 1073745153) : {
      | % START_R_7
      | }
  (junction 1073745153) -> (junction 1073745155) : {
      | }
  (junction 1073745155) -> (junction 1073745157)
  (junction 1073745157) -> (junction 1073745159) [order 1] : [(((t) >= (0) && (t) <= (20)))]
  (junction 1073745157) -> (junction 1073745165) [order 2]
  (junction 1073745159) -> (junction 1073745161) : {
      | reqtable_postcondition(((speed2)/120 < 1), 'R:1');
      |
      |
      |
      |
      | }
  (junction 1073745161) -> (junction 1073745163) : {
      | }
  (junction 1073745163) -> (junction 1073745165)
  (junction 1073745165) -> (junction 1073745167)
  (junction 1073745167) -> (junction 1073745169) : {
      | % END_R_7
      | }
  (junction 1073745169) -> (junction 1073745171) : {
      | % START_R_19
      | }
  (junction 1073745171) -> (junction 1073745173) : {
      | }
  (junction 1073745173) -> (junction 1073745175)
  (junction 1073745175) -> (junction 1073745177) [order 1] : [(((t) >= (0) && (t) <= (10)))]
  (junction 1073745175) -> (junction 1073745183) [order 2]
  (junction 1073745177) -> (junction 1073745179) : {
      | reqtable_postcondition(((RPM2)/4750 < 1), 'R:2');
      |
      |
      |
      |
      | }
  (junction 1073745179) -> (junction 1073745181) : {
      | }
  (junction 1073745181) -> (junction 1073745183)
  (junction 1073745183) -> (junction 1073745185)
  (junction 1073745185) -> (junction 1073745187) : {
      | % END_R_19
      | }
  (junction 1073745187) -> (junction 1073745189) : {
      | % START_R_34
      | }
  (junction 1073745189) -> (junction 1073745191) : {
      | }
  (junction 1073745191) -> (junction 1073745193)
  (junction 1073745193) -> (junction 1073745195) [order 1] : [((t)== 0)]
  (junction 1073745193) -> (junction 1073745201) [order 2]
  (junction 1073745195) -> (junction 1073745197) : {
      | flaga_out = true;
      | flagb_out = true;
      | flagc_out = true;
      |
      | }
  (junction 1073745197) -> (junction 1073745199) : {
      | }
  (junction 1073745199) -> (junction 1073745201)
  (junction 1073745201) -> (junction 1073745203)
  (junction 1073745203) -> (junction 1073745205) : {
      | % END_R_34
      | }
  (junction 1073745205) -> (junction 1073745207) : {
      | % START_R_22
      | }
  (junction 1073745207) -> (junction 1073745209) : {
      | }
  (junction 1073745209) -> (junction 1073745211)
  (junction 1073745211) -> (junction 1073745213) [order 1] : [(((t) <= (4))) && (speed1 >= 35)]
  (junction 1073745211) -> (junction 1073745219) [order 2]
  (junction 1073745213) -> (junction 1073745215) : {
      | flaga_out = false
      |
      |
      |
      | }
  (junction 1073745215) -> (junction 1073745217) : {
      | }
  (junction 1073745217) -> (junction 1073745219)
  (junction 1073745219) -> (junction 1073745221)
  (junction 1073745221) -> (junction 1073745223) : {
      | % END_R_22
      | }
  (junction 1073745223) -> (junction 1073745225) : {
      | % START_R_67
      | }
  (junction 1073745225) -> (junction 1073745227) : {
      | }
  (junction 1073745227) -> (junction 1073745229)
  (junction 1073745229) -> (junction 1073745231) [order 1] : [((t)> 4 || ((t)> 0 && speed1 < 35))]
  (junction 1073745229) -> (junction 1073745237) [order 2]
  (junction 1073745231) -> (junction 1073745233) : {
      | flaga_out = prev(flaga_out);
      |
      |
      |
      | }
  (junction 1073745233) -> (junction 1073745235) : {
      | }
  (junction 1073745235) -> (junction 1073745237)
  (junction 1073745237) -> (junction 1073745239)
  (junction 1073745239) -> (junction 1073745241) : {
      | % END_R_67
      | }
  (junction 1073745241) -> (junction 1073745243) : {
      | % START_R_52
      | }
  (junction 1073745243) -> (junction 1073745245) : {
      | }
  (junction 1073745245) -> (junction 1073745247)
  (junction 1073745247) -> (junction 1073745249) [order 1] : [duration((((t) <= (30))) && (RPM1 < 3000)) >= 30]
  (junction 1073745247) -> (junction 1073745255) [order 2]
  (junction 1073745249) -> (junction 1073745251) : {
      | reqtable_postcondition((((flaga_in) == (true))), 'R:6');
      |
      |
      |
      |
      | }
  (junction 1073745251) -> (junction 1073745253) : {
      | }
  (junction 1073745253) -> (junction 1073745255)
  (junction 1073745255) -> (junction 1073745257)
  (junction 1073745257) -> (junction 1073745259) : {
      | % END_R_52
      | }
  (junction 1073745259) -> (junction 1073745261) : {
      | % START_R_16
      | }
  (junction 1073745261) -> (junction 1073745263) : {
      | }
  (junction 1073745263) -> (junction 1073745265)
  (junction 1073745265) -> (junction 1073745267) [order 1] : [(((t) <= (8))) && (speed1 >= 50)]
  (junction 1073745265) -> (junction 1073745273) [order 2]
  (junction 1073745267) -> (junction 1073745269) : {
      |
      | flagb_out = false;
      |
      |
      | }
  (junction 1073745269) -> (junction 1073745271) : {
      | }
  (junction 1073745271) -> (junction 1073745273)
  (junction 1073745273) -> (junction 1073745275)
  (junction 1073745275) -> (junction 1073745277) : {
      | % END_R_16
      | }
  (junction 1073745277) -> (junction 1073745279) : {
      | % START_R_70
      | }
  (junction 1073745279) -> (junction 1073745281) : {
      | }
  (junction 1073745281) -> (junction 1073745283)
  (junction 1073745283) -> (junction 1073745285) [order 1] : [((t)> 8 || ((t)> 0 && speed1 < 50))]
  (junction 1073745283) -> (junction 1073745291) [order 2]
  (junction 1073745285) -> (junction 1073745287) : {
      |
      | flagb_out = prev(flagb_out);
      |
      |
      | }
  (junction 1073745287) -> (junction 1073745289) : {
      | }
  (junction 1073745289) -> (junction 1073745291)
  (junction 1073745291) -> (junction 1073745293)
  (junction 1073745293) -> (junction 1073745295) : {
      | % END_R_70
      | }
  (junction 1073745295) -> (junction 1073745297) : {
      | % START_R_55
      | }
  (junction 1073745297) -> (junction 1073745299) : {
      | }
  (junction 1073745299) -> (junction 1073745301)
  (junction 1073745301) -> (junction 1073745303) [order 1] : [duration((((t) <= (30))) && (RPM1 < 3000)) >= 30]
  (junction 1073745301) -> (junction 1073745309) [order 2]
  (junction 1073745303) -> (junction 1073745305) : {
      | reqtable_postcondition((((flagb_in) == (true))), 'R:9');
      |
      |
      |
      |
      | }
  (junction 1073745305) -> (junction 1073745307) : {
      | }
  (junction 1073745307) -> (junction 1073745309)
  (junction 1073745309) -> (junction 1073745311)
  (junction 1073745311) -> (junction 1073745313) : {
      | % END_R_55
      | }
  (junction 1073745313) -> (junction 1073745315) : {
      | % START_R_28
      | }
  (junction 1073745315) -> (junction 1073745317) : {
      | }
  (junction 1073745317) -> (junction 1073745319)
  (junction 1073745319) -> (junction 1073745321) [order 1] : [(((t) <= (20))) && (speed1 >= 65)]
  (junction 1073745319) -> (junction 1073745327) [order 2]
  (junction 1073745321) -> (junction 1073745323) : {
      |
      |
      | flagc_out = false;
      |
      | }
  (junction 1073745323) -> (junction 1073745325) : {
      | }
  (junction 1073745325) -> (junction 1073745327)
  (junction 1073745327) -> (junction 1073745329)
  (junction 1073745329) -> (junction 1073745331) : {
      | % END_R_28
      | }
  (junction 1073745331) -> (junction 1073745333) : {
      | % START_R_73
      | }
  (junction 1073745333) -> (junction 1073745335) : {
      | }
  (junction 1073745335) -> (junction 1073745337)
  (junction 1073745337) -> (junction 1073745339) [order 1] : [((t)> 20 || ((t)> 0 && speed1 < 65))]
  (junction 1073745337) -> (junction 1073745345) [order 2]
  (junction 1073745339) -> (junction 1073745341) : {
      |
      |
      | flagc_out = prev(flagc_out);
      |
      | }
  (junction 1073745341) -> (junction 1073745343) : {
      | }
  (junction 1073745343) -> (junction 1073745345)
  (junction 1073745345) -> (junction 1073745347)
  (junction 1073745347) -> (junction 1073745349) : {
      | % END_R_73
      | }
  (junction 1073745349) -> (junction 1073745351) : {
      | % START_R_58
      | }
  (junction 1073745351) -> (junction 1073745353) : {
      | }
  (junction 1073745353) -> (junction 1073745355)
  (junction 1073745355) -> (junction 1073745357) [order 1] : [duration((((t) <= (30))) && (RPM1 < 3000)) >= 30]
  (junction 1073745355) -> (junction 1073745363) [order 2]
  (junction 1073745357) -> (junction 1073745359) : {
      | reqtable_postcondition((((flagc_in) == (true))), 'R:12');
      |
      |
      |
      |
      | }
  (junction 1073745359) -> (junction 1073745361) : {
      | }
  (junction 1073745361) -> (junction 1073745363)
  (junction 1073745363) -> (junction 1073745365)
  (junction 1073745365) -> (junction 1073745367) : {
      | % END_R_58
      | }
  (junction 1073745367) -> (junction 1073745369) : {
      | % START_R_61
      | }
  (junction 1073745369) -> (junction 1073745371) : {
      | }
  (junction 1073745371) -> (junction 1073745373)
  (junction 1073745373) -> (junction 1073745375) [order 1] : [(((t) >= (0) && (t) <= (50)))]
  (junction 1073745373) -> (junction 1073745381) [order 2]
  (junction 1073745375) -> (junction 1073745377) : {
      | reqtable_postcondition((((speed2) >= (0))) && (((RPM2) >= (0))) && ((flaga_in)== true ||(flaga_in)== false) && ((flagb_in)== true ||(flagb_in)== false) && ((flagc_in)== true ||(flagc_in)== false), 'R:13');
      |
      |
      |
      |
      | }
  (junction 1073745377) -> (junction 1073745379) : {
      | }
  (junction 1073745379) -> (junction 1073745381)
  (junction 1073745381) -> (junction 1073745383)
  (junction 1073745383) -> (junction 1073745385) : {
      | % END_R_61
      | }
  data: RPM1 input; RPM2 input; speed1 input; speed2 input; flaga_out output boolean =true; flagc_out output boolean =true; flagb_out output boolean =true; flaga_in input boolean; flagc_in input boolean; flagb_in input boolean
